simulink model "gm_BlobAnalysisHDL"  (R2022b)
settings: Solver=FixedStepDiscrete  StartTime=0.0  StopTime=1/60  RelTol=1e-3
PreLoadFcn:
  | model_init_cca
InitFcn:
  | model_init_cca
undefined symbols (not defined in the file or in its folder): closenhood, gray, MaxBlobs, numCols, numRows, Rec, rgbmap24, SDTV, Ts
libraries: hdlsllib x37, simulink x21, hdlmdlgenlib x7, visionhdlutilities x5, visionhdlio x2, visiontextngfix x2, visionhdlmorphops x1, visionhdlconversions x1, visionsources x1, visiongeotforms x1
(part 3 of 3)

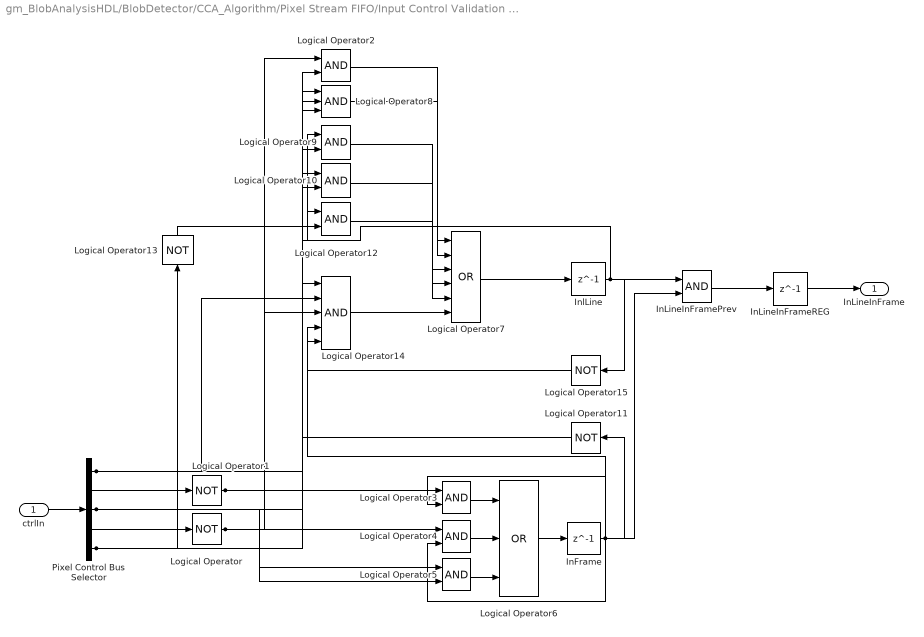
== system gm_BlobAnalysisHDL/BlobDetector/CCA_Algorithm/Pixel Stream FIFO/Input Control Validation /InLineInFrameTest ==
  ctrlIn : Inport
  InFrame : Delay  DelayLength=1
  InLineInFramePrev : Logic  AllPortsSameDT=off  OutDataTypeStr=boolean
  InLineInFrameREG : Delay  DelayLength=1
  InlLine : Delay  DelayLength=1
  Logical Operator{,1,11,13,15} (5 alike) : Logic  Operator=NOT  AllPortsSameDT=off  OutDataTypeStr=boolean
  Logical Operator{2..5,9..10,12} (7 alike) : Logic  AllPortsSameDT=off  OutDataTypeStr=boolean
  Logical Operator14 : Logic  Inputs=5  AllPortsSameDT=off  OutDataTypeStr=boolean
  Logical Operator6 : Logic  Operator=OR  Inputs=3  AllPortsSameDT=off  OutDataTypeStr=boolean
  Logical Operator7 : Logic  Operator=OR  Inputs=6  AllPortsSameDT=off  OutDataTypeStr=boolean
  Logical Operator8 : Logic  Inputs=3  AllPortsSameDT=off  OutDataTypeStr=boolean
  Pixel Control Bus Selector : BusSelector  OutputSignals=hStart,hEnd,vStart,vEnd,valid
  InLineInFrame : Outport  SampleTime=1.2796101795549e-07  VectorParamsAs1DForOutWhenUnconnected=off
  wires:
  InFrame/1 -> Logical Operator11/1, InLineInFramePrev/2, Logical Operator4/2, Logical Operator3/2, Logical Operator14/4
  InLineInFramePrev/1 -> InLineInFrameREG/1
  InLineInFrameREG/1 -> InLineInFrame/1
  InlLine/1 -> InLineInFramePrev/1, Logical Operator9/1, Logical Operator2/2, Logical Operator15/1, Logical Operator12/1, Logical Operator10/2
  Logical Operator/1 -> Logical Operator4/1, Logical Operator14/3
  Logical Operator1/1 -> Logical Operator3/1, Logical Operator2/1
  Logical Operator11/1 -> Logical Operator10/1
  Logical Operator13/1 -> Logical Operator12/2
  Logical Operator5/1 -> Logical Operator6/3
  Logical Operator8/1 -> Logical Operator7/2
  Pixel Control Bus Selector/1 -> Logical Operator8/2, Logical Operator14/2
  Pixel Control Bus Selector/2 -> Logical Operator1/1
  Pixel Control Bus Selector/3 -> Logical Operator8/3, Logical Operator5/2, Logical Operator9/2
  Pixel Control Bus Selector/4 -> Logical Operator/1
  Pixel Control Bus Selector/5 -> Logical Operator8/1, Logical Operator5/1, Logical Operator13/1, Logical Operator14/1
  ctrlIn/1 -> Pixel Control Bus Selector/1
  Logical Operator6/1 -> InFrame/1
  Logical Operator4/1 -> Logical Operator6/2
  Logical Operator3/1 -> Logical Operator6/1
  Logical Operator7/1 -> InlLine/1
  Logical Operator14/1 -> Logical Operator7/6
  Logical Operator15/1 -> Logical Operator14/5
  Logical Operator12/1 -> Logical Operator7/5
  Logical Operator10/1 -> Logical Operator7/4
  Logical Operator9/1 -> Logical Operator7/3
  Logical Operator2/1 -> Logical Operator7/1

== system gm_BlobAnalysisHDL/BlobDetector/CCA_Algorithm/cca/Merge/Hold Signal ==
  triggerStart : Inport  OutDataTypeStr=boolean  PortDimensions=1  SampleTime=1.2796101795549e-07
  triggerEnd : Inport  Port=2  OutDataTypeStr=boolean  PortDimensions=1  SampleTime=1.2796101795549e-07
  Constant5 : Constant  Value=0  OutDataTypeStr=boolean  SampleTime=-1
  Constant6 : Constant  OutDataTypeStr=boolean  SampleTime=-1
  Delay6 : Delay  DelayLength=1  InitialCondition=0  UseCircularBuffer=on
  Logical Operator : Logic  IconShape=distinctive  AllPortsSameDT=off  OutDataTypeStr=boolean
  Logical Operator1 : Logic  Operator=NOT  IconShape=distinctive  AllPortsSameDT=off  OutDataTypeStr=boolean
  Switch3 : Switch  Criteria=u2 ~= 0  SaturateOnIntegerOverflow=off  InputSameDT=off
  Switch4 : Switch  Criteria=u2 ~= 0  SaturateOnIntegerOverflow=off  InputSameDT=off
  Signal : Outport  SampleTime=1.2796101795549e-07  VectorParamsAs1DForOutWhenUnconnected=off
  wires:
  Constant5/1 -> Switch3/1
  Constant6/1 -> Switch4/1
  Logical Operator/1 -> Switch3/2
  Logical Operator1/1 -> Logical Operator/2
  Switch3/1 -> Signal/1, Delay6/1
  triggerStart/1 -> Logical Operator1/1, Switch4/2
  triggerEnd/1 -> Logical Operator/1
  Switch4/1 -> Switch3/3
  Delay6/1 -> Switch4/3

== system gm_BlobAnalysisHDL/BlobDetector/CCA_Algorithm/cca/Merge/counterTrigger ==
  triggerStart : Inport  OutDataTypeStr=boolean  PortDimensions=1  SampleTime=1.2796101795549e-07
  suppress : Inport  Port=2  OutDataTypeStr=boolean  PortDimensions=1  SampleTime=1.2796101795549e-07
  Compare To Constant : simulink/Logic and Bit Operations/Compare To Constant  relop===  const="fi(0,0,8,0,\"hex\",\"03\")"  OutDataTypeStr=boolean
  Constant : Constant  OutDataTypeStr=uint8  SampleTime=1.2796101795549e-07
  Constant5 : Constant  Value=0  OutDataTypeStr=uint8  SampleTime=1.2796101795549e-07
  Constant6 : Constant  OutDataTypeStr=fixdt(0, 9, 0)  SampleTime=1.2796101795549e-07
  Delay6 : Delay  DelayLength=double(1)  InitialCondition=0  SampleTime=1.2796101795549e-07
  Logical Operator : Logic  AllPortsSameDT=off  OutDataTypeStr=boolean  SampleTime=1.2796101795549e-07
  Logical Operator1 : Logic  Operator=NOT  Inputs=1  AllPortsSameDT=off  OutDataTypeStr=boolean  SampleTime=1.2796101795549e-07
  Sum : Sum  AccumDataTypeStr=fixdt(0, 9, 0)  OutDataTypeStr=fixdt(0, 9, 0)  SampleTime=1.2796101795549e-07
  Switch3 : Switch  Criteria=u2 ~= 0  Threshold=double(0)  OutDataTypeStr=uint8  SampleTime=1.2796101795549e-07  SaturateOnIntegerOverflow=off  InputSameDT=off
  Switch4 : Switch  Criteria=u2 ~= 0  Threshold=double(0)  OutDataTypeStr=fixdt(0, 9, 0)  SampleTime=1.2796101795549e-07  SaturateOnIntegerOverflow=off  InputSameDT=off
  Signal : Outport  SampleTime=1.2796101795549e-07  VectorParamsAs1DForOutWhenUnconnected=off
  wires:
  Compare To Constant/1 -> Signal/1
  Constant/1 -> Sum/2
  Constant5/1 -> Switch3/1
  Constant6/1 -> Switch4/1
  Logical Operator/1 -> Switch3/2
  Logical Operator1/1 -> Logical Operator/2
  Switch3/1 -> Compare To Constant/1, Sum/1
  triggerStart/1 -> Logical Operator1/1, Switch4/2
  suppress/1 -> Logical Operator/1
  Sum/1 -> Delay6/1
  Switch4/1 -> Switch3/3
  Delay6/1 -> Switch4/3

== system gm_BlobAnalysisHDL/BlobDetector/CCA_Algorithm/cca/accum_to_pos/Data Type Conversion2 ==
  In1 : Inport
  Data Type Conversion2 : DataTypeConversion  OutDataTypeStr=fixdt(0, 32, 30)  SampleTime=1.2796101795549e-07  SaturateOnIntegerOverflow=off  RndMeth=Floor
  Data Type Conversion2_pd1 : Delay  DelayLength=6
  Out1 : Outport
  wires:
  In1/1 -> Data Type Conversion2/1
  Data Type Conversion2/1 -> Data Type Conversion2_pd1/1
  Data Type Conversion2_pd1/1 -> Out1/1

== system gm_BlobAnalysisHDL/BlobDetector/CCA_Algorithm/cca/accum_to_pos/Data Type Conversion3 ==
  In1 : Inport
  Data Type Conversion3 : DataTypeConversion  OutDataTypeStr=single  SampleTime=1.2796101795549e-07  SaturateOnIntegerOverflow=off  RndMeth=Floor
  Data Type Conversion3_pd1 : Delay  DelayLength=6
  Out1 : Outport
  wires:
  In1/1 -> Data Type Conversion3/1
  Data Type Conversion3/1 -> Data Type Conversion3_pd1/1
  Data Type Conversion3_pd1/1 -> Out1/1

== system gm_BlobAnalysisHDL/BlobDetector/CCA_Algorithm/cca/accum_to_pos/Math Reciprocal1 ==
  In1 : Inport
  Math Reciprocal1 : Math  Operator=reciprocal  SampleTime=1.2796101795549e-07
  Math Reciprocal1_pd1 : Delay  DelayLength=31
  Out1 : Outport
  wires:
  In1/1 -> Math Reciprocal1/1
  Math Reciprocal1/1 -> Math Reciprocal1_pd1/1
  Math Reciprocal1_pd1/1 -> Out1/1

== system gm_BlobAnalysisHDL/BlobDetector/CCA_Algorithm/cca/bbox_store/resolve ==
  fromRAM : Inport  OutDataTypeStr=fixdt(0, 34, 0)  PortDimensions=1  SampleTime=1.2796101795549e-07
  bbox : Inport  Port=2  OutDataTypeStr=fixdt(0, 34, 0)  PortDimensions=1  SampleTime=1.2796101795549e-07
  Bit Concat : hdlsllib/Logic and Bit Operations/Bit Concat  numInputs=4
  Compare To Zero : simulink/Logic and Bit Operations/Compare To Zero  relop===  OutDataTypeStr=boolean
  Relational Operator : RelationalOperator  Operator=<  OutDataTypeStr=boolean  InputSameDT=off
  Relational Operator1 : RelationalOperator  Operator=<  OutDataTypeStr=boolean  InputSameDT=off
  Relational Operator2 : RelationalOperator  Operator=>  OutDataTypeStr=boolean  InputSameDT=off
  Relational Operator3 : RelationalOperator  Operator=>  OutDataTypeStr=boolean  InputSameDT=off
  Switch{,1..4} (5 alike) : Switch  Criteria=u2 ~= 0  SaturateOnIntegerOverflow=off  InputSameDT=off
  splitBBoxNEW : Subsystem
  splitBBoxRAM : Subsystem
  toRAM : Outport  SampleTime=1.2796101795549e-07  VectorParamsAs1DForOutWhenUnconnected=off
  wires:
  Bit Concat/1 -> Switch4/3
  Compare To Zero/1 -> Switch4/2
  Relational Operator/1 -> Switch/2
  Relational Operator1/1 -> Switch1/2
  Relational Operator2/1 -> Switch2/2
  Relational Operator3/1 -> Switch3/2
  Switch/1 -> Bit Concat/1
  Switch1/1 -> Bit Concat/2
  Switch2/1 -> Bit Concat/3
  Switch3/1 -> Bit Concat/4
  Switch4/1 -> toRAM/1
  splitBBoxNEW/1(X1) -> Switch/3, Relational Operator/2
  splitBBoxNEW/2(Y1) -> Switch1/3, Relational Operator1/2
  splitBBoxNEW/3(X2) -> Switch2/3, Relational Operator2/2
  splitBBoxNEW/4(Y2) -> Switch3/3, Relational Operator3/2
  splitBBoxRAM/1(X1) -> Switch/1, Relational Operator/1
  splitBBoxRAM/2(Y1) -> Switch1/1, Relational Operator1/1
  splitBBoxRAM/3(X2) -> Switch2/1, Relational Operator2/1
  splitBBoxRAM/4(Y2) -> Switch3/1, Relational Operator3/1
  fromRAM/1 -> Compare To Zero/1, splitBBoxRAM/1(In1)
  bbox/1 -> Switch4/1, splitBBoxNEW/1(In1)

== system gm_BlobAnalysisHDL/BlobDetector/CCA_Algorithm/cca/bbox_store/resolve/splitBBoxNEW ==
  In1 : Inport  OutDataTypeStr=fixdt(0, 34, 0)  PortDimensions=1  SampleTime=1.2796101795549e-07
  Bit Slice4 : hdlsllib/Logic and Bit Operations/Bit Slice  lidx=ceil(log2(numRows))-1  ridx=0
  Bit Slice5 : hdlsllib/Logic and Bit Operations/Bit Slice  lidx=ceil(log2(numRows))+ceil(log2(numCols))-1  ridx=ceil(log2(numRows))
  Bit Slice6 : hdlsllib/Logic and Bit Operations/Bit Slice  lidx=2*ceil(log2(numRows))+ceil(log2(numCols))-1  ridx=ceil(log2(numRows))+ceil(log2(numCols))
  Bit Slice7 : hdlsllib/Logic and Bit Operations/Bit Slice  lidx=2*ceil(log2(numRows))+2*ceil(log2(numCols))-1  ridx=2*ceil(log2(numRows))+ceil(log2(numCols))
  X1 : Outport  SampleTime=1.2796101795549e-07  VectorParamsAs1DForOutWhenUnconnected=off
  Y1 : Outport  Port=2  SampleTime=1.2796101795549e-07  VectorParamsAs1DForOutWhenUnconnected=off
  X2 : Outport  Port=3  SampleTime=1.2796101795549e-07  VectorParamsAs1DForOutWhenUnconnected=off
  Y2 : Outport  Port=4  SampleTime=1.2796101795549e-07  VectorParamsAs1DForOutWhenUnconnected=off
  wires:
  Bit Slice4/1 -> Y2/1
  Bit Slice5/1 -> X2/1
  Bit Slice6/1 -> Y1/1
  Bit Slice7/1 -> X1/1
  In1/1 -> Bit Slice7/1, Bit Slice6/1, Bit Slice5/1, Bit Slice4/1

== system gm_BlobAnalysisHDL/BlobDetector/CCA_Algorithm/cca/bbox_store/resolve/splitBBoxRAM ==
  In1 : Inport  OutDataTypeStr=fixdt(0, 34, 0)  PortDimensions=1  SampleTime=1.2796101795549e-07
  Bit Slice4 : hdlsllib/Logic and Bit Operations/Bit Slice  lidx=ceil(log2(numRows))-1  ridx=0
  Bit Slice5 : hdlsllib/Logic and Bit Operations/Bit Slice  lidx=ceil(log2(numRows))+ceil(log2(numCols))-1  ridx=ceil(log2(numRows))
  Bit Slice6 : hdlsllib/Logic and Bit Operations/Bit Slice  lidx=2*ceil(log2(numRows))+ceil(log2(numCols))-1  ridx=ceil(log2(numRows))+ceil(log2(numCols))
  Bit Slice7 : hdlsllib/Logic and Bit Operations/Bit Slice  lidx=2*ceil(log2(numRows))+2*ceil(log2(numCols))-1  ridx=2*ceil(log2(numRows))+ceil(log2(numCols))
  X1 : Outport  SampleTime=1.2796101795549e-07  VectorParamsAs1DForOutWhenUnconnected=off
  Y1 : Outport  Port=2  SampleTime=1.2796101795549e-07  VectorParamsAs1DForOutWhenUnconnected=off
  X2 : Outport  Port=3  SampleTime=1.2796101795549e-07  VectorParamsAs1DForOutWhenUnconnected=off
  Y2 : Outport  Port=4  SampleTime=1.2796101795549e-07  VectorParamsAs1DForOutWhenUnconnected=off
  wires:
  Bit Slice4/1 -> Y2/1
  Bit Slice5/1 -> X2/1
  Bit Slice6/1 -> Y1/1
  Bit Slice7/1 -> X1/1
  In1/1 -> Bit Slice7/1, Bit Slice6/1, Bit Slice5/1, Bit Slice4/1

== matlab function gm_BlobAnalysisHDL/BlobDetector/CCA_Algorithm/Pixel Stream FIFO/CastIfBoolean/visionhdlutilities_c1_CastIfBoolean ==
  data: u input; y output
function y = CastIfBoolean(u)

% Copyright 2017-2021 The MathWorks, Inc.

%#codegen

if islogical(u)
    y = fi(u,0,1,0);
else 
    y = u;
end

== matlab function gm_BlobAnalysisHDL/BlobDetector/CCA_Algorithm/Pixel Stream FIFO/Memory Controller/visionhdlutilities_c2_Memory_Controller ==
  data: hEnd input; pop output; readCountIn input; writeCountLimit input; vStart input
function pop = MemoryController(hEnd, readCountIn, writeCountLimit, vStart)

% Copyright 2017-2021 The MathWorks, Inc.

%#codegen

persistent BufferState;

S0 = fi(0,0,1,0);
S1 = fi(1,0,1,0);

if isempty(BufferState)
    BufferState = S0;
end

switch BufferState

    case S0 %%% Idle State
        pop = false;
        if hEnd
            BufferState = S1;
        else
            BufferState = S0;
        end

    case S1 %%% Pop until limit reached
        pop = true;
        if readCountIn == writeCountLimit || vStart
            BufferState = S0;
        else
            BufferState = S1;
        end

    otherwise
        pop = false;

end

== matlab function gm_BlobAnalysisHDL/BlobDetector/CCA_Algorithm/Pixel Stream FIFO/ReshapeFunction/visionhdlutilities_c3_ReshapeFunction ==
  data: u input; y output; v input
function y = fcn(u,v)

% Copyright 2017-2021 The MathWorks, Inc.

%#codegen
y = reshape(u,size(v,1),size(v,2));
end

== matlab function gm_BlobAnalysisHDL/readCCADataOut ==
  data: rdy input; rdidx output; wridx output; wrvalue output; num2rd input; fbidx input; wrenb output; maxnumblobs parameter
function [rdidx, wridx, wrvalue, wrenb]  = fcn(rdy, num2rd, fbidx, maxnumblobs)

IDLE     = 0;
READNEXT = 1;
WAIT     = 2;
ACTIVE   = 3;
ZEROOUT  = 4;

persistent state rdidxreg num2rdreg wridxreg
if isempty(state)
    state = IDLE;
    num2rdreg = uint16(0);
    rdidxreg = uint16(1);
    wridxreg = uint16(1);  % limit number to 2^16
end
wrvalue = false;
wrenb = false;

switch state
    case IDLE
        rdidxreg(:) = 0;
        if rdy == true % && num2rd > 0
            state = WAIT;
            rdidxreg(:) = 1;  % start at 1 to compare to 1 instead of 0
            wridxreg(:) = 1;  % one-based assignment index
            num2rdreg(:) = num2rd;  % num to read this frame
        end        
    case READNEXT
        if rdidxreg < num2rdreg
            rdidxreg(:) = rdidxreg + 1;
            state = WAIT;
        else
            state = ZEROOUT;
        end
    case WAIT
        % wait while rdidx not equal to feedback index
        if rdidxreg == uint16(fbidx)
            state = ACTIVE;
        end
    case ACTIVE
         state = READNEXT;
         wridxreg(:) = wridxreg + 1;
         wrvalue = true;  % Write the value provided
         wrenb = true; % enable the write
    case ZEROOUT
        % write zeros to the rest of the entries
         wridxreg(:) = wridxreg + 1;
         wrvalue = false;  % RESET the value entry
         wrenb = true; % enable the write
         if wridxreg == maxnumblobs
             state = IDLE;
         end
end

rdidx = rdidxreg;
wridx = wridxreg;

== matlab function gm_BlobAnalysisHDL/BlobDetector/CCA_Algorithm/cca/ReadBlobs/ReadBlobs ==
  data: start input; blobIdx output; maxIdx input; valid output; skipidx input; rdreset output boolean; MaxBlobs parameter; numFnd output
function [blobIdx, valid, rdreset, numFnd] = readblobdata(start, maxIdx, skipidx, MaxBlobs)
%#codegen

IDLE = fi(0,0,3,0);
WAIT = fi(1,0,3,0);
NEXT = fi(3,0,3,0);

persistent state index numFndIncr validreg rdresetreg
if isempty(index)
    state = IDLE;
    index = fi(0,0,ceil(log2(MaxBlobs)),0);
    numFndIncr = uint16(0);
    validreg = false;
    rdresetreg = false;
end

blobIdx = index;
numFnd = numFndIncr;
valid = validreg;
rdreset = rdresetreg;

switch state
    case IDLE
        index(:) = 0;
        rdresetreg = false;
        validreg = false;
        if start
            index(:) = 1;
            state = WAIT;
            rdresetreg = true;
            numFndIncr(:) = 0;
        end
    case WAIT
        state = NEXT;
        index(:) = index + 1;        
    case NEXT
        validreg = false;
        if skipidx == 0
            validreg = true;
            numFndIncr(:) = numFndIncr + 1;
        end        
        if index > maxIdx
            state = IDLE;
        end
        index(:) = index + 1;        
end

== matlab function gm_BlobAnalysisHDL/BlobDetector/CCA_Algorithm/cca/labelandmerge/labelandmerge ==
  data: pixIn input; ctrlIn input; newLabel output fixdt(0,ceil(log2(MaxBlobs)),0); labelAbove input fixdt(0,ceil(log2(MaxBlobs)),0); labelAboveLeft input; labelAboveRight input; rst input; mergeIndxs output; maxIdx output; MaxBlobs parameter
function [newLabel, mergeIndxs, maxIdx] = fcn(pixIn, ctrlIn, labelAbove, labelAboveLeft, labelAboveRight, rst,  MaxBlobs)
%#codegen

persistent nextLabel newLabelReg mergeIndxsReg beforeLabel mergeIndxsRegLast

if isempty(nextLabel)
    nextLabel = fi(1,0,ceil(log2(MaxBlobs)),0); % uint16(1);
    beforeLabel = fi(1,0,ceil(log2(MaxBlobs)),0); % uint16(1);
    newLabelReg = fi(0,0,ceil(log2(MaxBlobs)),0); % uint16(0);
    mergeIndxsReg = fi(0,0,32,0);
    mergeIndxsRegLast = fi(0,0,32,0);
    %numBlobsReg = uint32(0);
end

newLabel = newLabelReg;
mergeIndxs = uint32(mergeIndxsReg);
maxIdx = nextLabel-1;
% numBlobs = numBlobsReg;

beforeLabel = newLabelReg;

newLabelReg(:) = 0;
mergeIndxsReg(:) = 0;

if rst
    nextLabel(:) = 1;
    beforeLabel(:) = 0;
    %numBlobsReg(:) = 0;
end

if ctrlIn.hStart
    mergeIndxsRegLast(:) = 0;
end

if pixIn && ctrlIn.valid
% assign new value by priority - LAST < ABOVE < NEW
    if beforeLabel ~= 0
        % look for label on the same line just before
        newLabelReg = beforeLabel;
        % check to see if we need to merge
        if labelAbove ~= 0 && (beforeLabel ~= labelAbove)
                mergeIndxsReg = bitconcat(fi(labelAbove,0,16,0), fi(beforeLabel,0,16,0));
                if(mergeIndxsReg == mergeIndxsRegLast)
                    mergeIndxsReg(:) = 0;
                else
                    mergeIndxsRegLast = mergeIndxsReg;
                    %numBlobsReg(:) = numBlobsReg - 1;
                end
        elseif labelAboveRight ~= 0 && (beforeLabel ~= labelAboveRight) 
                mergeIndxsReg = bitconcat(fi(labelAboveRight,0,16,0), fi(beforeLabel,0,16,0));
                if(mergeIndxsReg == mergeIndxsRegLast)
                    mergeIndxsReg(:) = 0;
                else
                    mergeIndxsRegLast = mergeIndxsReg;
                    %numBlobsReg(:) = numBlobsReg - 1;
                end
        end
    elseif labelAbove ~= 0
        % look for label in the same column just above
        newLabelReg(:) = labelAbove;
        % check to see if already merged on this same line
        if mergeIndxsRegLast ~= 0
            labelAboveMerged = bitsliceget(mergeIndxsRegLast,32,17);
            if labelAbove == labelAboveMerged
                newLabelReg(:) = bitsliceget(mergeIndxsRegLast,16,1);
            end            
        end
    elseif labelAboveLeft ~= 0 
        % look for label in the same column just above and to the left
        newLabelReg(:) = labelAboveLeft;
        % check to see if already merged on this same line
        if mergeIndxsRegLast ~= 0
            labelAboveMerged = bitsliceget(mergeIndxsRegLast,32,17);
            if labelAboveLeft == labelAboveMerged
                newLabelReg(:) = bitsliceget(mergeIndxsRegLast,16,1);
            end            
        end
    elseif labelAboveRight ~= 0 
        % look for label in the same column just above and to the left
        newLabelReg(:) = labelAboveRight;
        % check to see if already merged on this same line
        if mergeIndxsRegLast ~= 0
            labelAboveMerged = bitsliceget(mergeIndxsRegLast,32,17);
            if labelAboveRight == labelAboveMerged
                newLabelReg(:) = bitsliceget(mergeIndxsRegLast,16,1);
            end            
        end
    else
        % else just assign a new label
        newLabelReg = nextLabel;
        if nextLabel == uint16(MaxBlobs-1)
            nextLabel(:) = 1;
        else
            nextLabel(:) = nextLabel + 1;
        end        
        %numBlobsReg(:) = numBlobsReg + 1;
    end
end
